simulink model "VdP_CL_sim"  (R2023b)
settings: Solver=ode4  StartTime=0.0  StopTime=Tf  FixedStep=Ts  RelTol=1e-3
values from neighbouring files (symbols this model uses):
  Kc = [-2 -5]    [VdP_CL.m]
  t_start = 20    [VdP_CL.m]    (also in VdP_RCAC_ESC.m)
  x0 = [1;0]    [VdP_CL.m]    (also in VdP_RCAC_ESC.m)
settings Model: Creator=Juan Augusto Paredes  LastModifiedBy=Juan Augusto Paredes

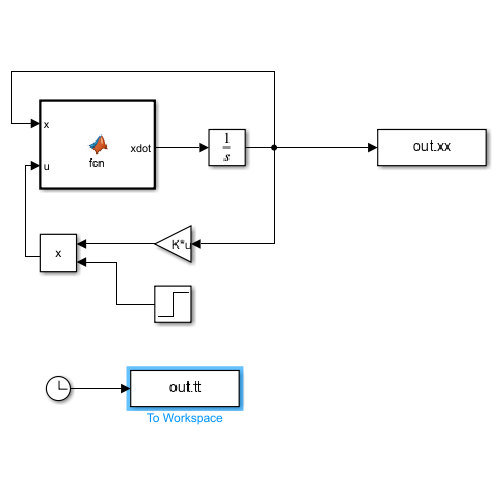
[thumbnail: Simulink's stored preview of the top-level diagram]
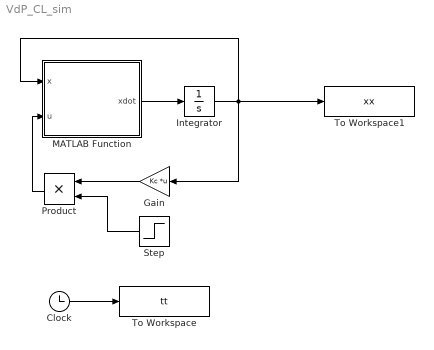
== system VdP_CL_sim ==
  Clock : Clock
  Gain : Gain  Gain=Kc  Multiplication=Matrix(K*u)
  Integrator : Integrator  InitialCondition=x0
  MATLAB Function : MATLAB Function  TreatAsAtomicUnit=on
  Product : Product
  Step : Step  Time=t_start  SampleTime=0
  To Workspace : ToWorkspace  VariableName=tt  SampleTime=-1
  To Workspace1 : ToWorkspace  VariableName=xx  SampleTime=-1
  wires:
  MATLAB Function/1(xdot) -> Integrator/1
  Integrator/1 -> To Workspace1/1, MATLAB Function/1(x), Gain/1
  Gain/1 -> Product/1
  Product/1 -> MATLAB Function/2(u)
  Step/1 -> Product/2
  Clock/1 -> To Workspace/1

== matlab function VdP_CL_sim/MATLAB Function ==
  data: x input size=2; u input size=1; xdot output size=2
function xdot = fcn(x,u)

xdot = [x(2) ;...
        -x(1) - ((x(2))^2 - 1)*x(2) + u];

end
